simulink subsystem "PvtSubSys_LSM"  (R2020b)
settings: Solver=VariableStepAuto  StartTime=0.0  StopTime=10.0  RelTol=1e-3
values from neighbouring files (symbols this model uses):
  P_LSM_ALC_Enable = 0.0    [LSM_Parameter.sldd]
  P_LSM_DOP_C0_EN_Limit = 0.8    [LSM_Parameter.sldd]
  P_LSM_DOP_C0_out_Limit = 2.0    [LSM_Parameter.sldd]
  P_LSM_DOP_C1_EN_Limit : value not decoded    [LSM_Parameter.sldd]
  P_LSM_DOP_C1_out_Limit : value not decoded    [LSM_Parameter.sldd]
  P_LSM_DOP_C1AndC2_Lim_X : value not decoded    [LSM_Parameter.sldd]
  P_LSM_DOP_C2_EN_Limit : value not decoded    [LSM_Parameter.sldd]
  P_LSM_DOP_C2_out_Limit : value not decoded    [LSM_Parameter.sldd]
  P_LSM_DOP_In_Pre2Dop_Dis = 1.0    [LSM_Parameter.sldd]
  P_LSM_DOP_Out_Pre2Dop_Dis = 2.0    [LSM_Parameter.sldd]
  P_LSM_DOP_PreDis_X : value not decoded    [LSM_Parameter.sldd]
  P_LSM_DOP_PreDis_Y : value not decoded    [LSM_Parameter.sldd]
  P_LSM_DOPValid_CheckTime = 0.06    [LSM_Parameter.sldd]
  P_LSM_DoubleLine_Curr2Cent_Dislimit = 0.5    [LSM_Parameter.sldd]
  P_LSM_DoubleLine_Dop2Cent_Dislimit = 0.5    [LSM_Parameter.sldd]
  P_LSM_DoubleLine_DOPOut_C1 : value not decoded    [LSM_Parameter.sldd]
  P_LSM_DoubleLine_Pre2Cent_Dislimit = 1.0    [LSM_Parameter.sldd]
  P_LSM_IFV2CenterAxis = 0.0    [LSM_Parameter.sldd]
  P_LSM_IFV2RearAxis = 0.0    [LSM_Parameter.sldd]
  P_LSM_LineSTD_Limit = 0.15    [LSM_Parameter.sldd]
  P_LSM_NOH_Switch = 0.0    [LSM_Parameter.sldd]
  P_LSM_Pre_t = 0.0    [LSM_Parameter.sldd]
  P_LSM_SingleLine_Cent2Edge_Dislimit = 100.0    [LSM_Parameter.sldd]
  P_LSM_SingleLine_Curr2Cent_Dislimit = 0.2    [LSM_Parameter.sldd]
  P_LSM_SingleLine_Dop2Cent_Dislimit = 0.2    [LSM_Parameter.sldd]
  P_LSM_SingleLine_DOPOut_C1 : value not decoded    [LSM_Parameter.sldd]
  P_LSM_SingleLine_Pre2Cent_Dislimit = 0.5    [LSM_Parameter.sldd]
undefined symbols (not defined in the file or in its folder): P_LSM_LineWijCal_C12, P_LSM_LineWijCal_C13, P_LSM_PosLineLcFac
libraries: simulink x92, TrueDurationTime x2
(part 1 of 9)
settings Model: Creator=GW00232905  LastModifiedBy=GW00232905

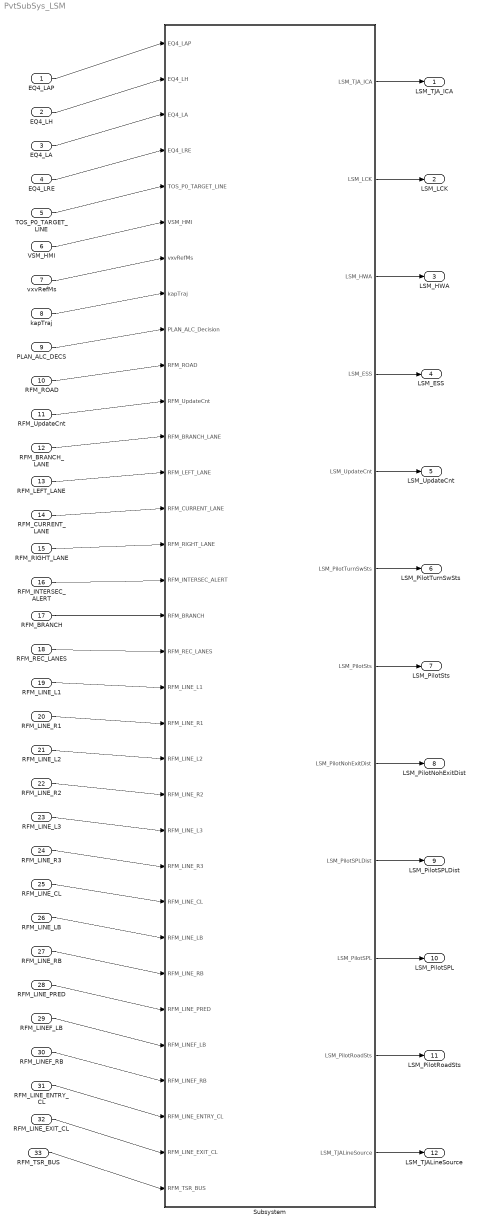
== system PvtSubSys_LSM ==
  EQ4_LAP : Inport  Description=预留  OutDataTypeStr=Bus: EQ4_LAP_BUS  PortDimensions=1  BusOutputAsStruct=on
  EQ4_LH : Inport  Description=|  Port=2  OutDataTypeStr=Bus: EQ4_LH_BUS  PortDimensions=1  BusOutputAsStruct=on
      | LH_Sync_ID	 	uint8		|		判断主车道线是否更新
      | LA_Lanes_Count		uint8		|		主车道线数量
      | LH_Availability_Stat  	uint8		|		主车道线是否可用
      | LH_Line_First_C0		single		m		主车道线第一段参数C0;曲线方程：y=c0+c1*x+c2*x^2+c3*x^3;
      | LH_Line_First_C1	         single		rad		主车道线第一段参数C1
      | LH_Line_First_C2	         single		1/m		主车道线第一段参数C2
      | LH_Line_First_C3	         single		1/m^2		主车道线第一段参数C3
      | LH_First_VR_Start	         single		m		主车道线第一段有效范围起点
      | LH_First_VR_End	         single		m		主车道线第一段有效范围终点
      | LH_lanemark_Type	         uint8		|		主车道线标记类型分类(实线，虚线等)
      | LH_DLM_Type	         uint8		|		主车道线双车道线标志
      | LH_Side	                   uint8		|		主车道线边界
      | LH_Marker_Width	         single		m		主车道线宽度
      | LH_Crossing	         uint8		|		判断是否跨越车道线
      | LH_Confidence	         uint8		|		主车道线置信度
      | LH_Color	                   uint8		|		主车道线颜色
      | LH_Line_Second_C0	          single		m		主车道线第二段参数C0;曲线方程：y=c0+c1*x+c2*x^2+c3*x^3
      | LH_Line_Second_C1	          single		rad		主车道线第二段参数C1
      | LH_Line_Second_C2	          single		1/m		主车道线第二段参数C2
      | LH_Line_Second_C3	          single		1/m^2		主车道线第二段参数C3
      | LH_Second_VR_Start	          single		m		主车道线第二段有效范围起点
      | LH_Second_VR_End	          single		m		主车道线第二段有效范围终点
  EQ4_LA : Inport  Description=|  Port=3  OutDataTypeStr=Bus: EQ4_LA_BUS  PortDimensions=1  BusOutputAsStruct=on
      | LA_Sync_ID		uint8		|		判断邻车道线是否更新
      | LA_Adjacent_Count		uint8		|		邻车道线数量		
      | LA_Availability_State	uint8		|		车道边界是否可用
      | LA_Line_C0		single		m		邻车道参数C0;曲线方程：y=c0+c1*x+c2*x^2+c3*x^3;
      | LA_Line_C1		single		rad		邻车道参数C1
      | LA_Line_C2		single		1/m		邻车道参数C2
      | LA_Line_C3		single		1/m^2		邻车道参数C3
      | LA_View_Range_Start	single		m		邻车道线有效范围起点
      | LA_View_Range_End	         single		m		邻车道线有效范围终点
      | LA_Lanemark_Type		uint8		|		邻车道线标记类型分类（实线，虚线等）
      | LA_DLM_Type		uint8		|		邻车道线双车道线标志
      | LA_Line_Side		uint8		|		车道标志相对于主车道的作用
      | LA_Marker_Width		single		m		车道线宽度
      | LA_Confidence		uint8		|		车道标志的置信度
  EQ4_LRE : Inport  Description=|  Port=4  OutDataTypeStr=Bus: EQ4_LRE_BUS  PortDimensions=1  BusOutputAsStruct=on
      | LRE_Sync_ID		uint8		|		判断边界车道线是否更新
      | LRE_Count		          uint8		|		边界车道线数量			
      | LRE_AvaiLREbility_State	uint8		|		边界车道线是否可用
      | LRE_Line_C0		single		m		边界车道线参数C0;曲线方程：y=c0+c1*x+c2*x^2+c3*x^3;
      | LRE_Line_C1		single		rad		边界车道线参数C1
      | LRE_Line_C2		single		1/m		边界车道线参数C2
      | LRE_Line_C3		single		1/m^2		边界车道线参数C3
      | LRE_View_Range_Start	single		m		边界车道线有效范围起点
      | LRE_View_Range_End	         single		m		边界车道线有效范围终点
      | LRE_Side			uint8		|		边界车道线标记
      | LRE_Confidence		uint8		|		边界车道线置信度
  TOS_P0_TARGET_LINE : Inport  Description=|  Port=5  OutDataTypeStr=Bus: TOS_P0_TARGET_LINE_BUS  PortDimensions=1  BusOutputAsStruct=on
      | OTL_Valid     uint8     |       OTL是否有效
      | OTL_C3        single    1/m^2   OTL参数C3;曲线方程：y=c0+c1*x+c2*x^2+c3*x^3
      | OTL_C2        single    1/m     OTL参数C2
      | OTL_C1        single    rad     OTL参数C1
      | OTL_C0        single    m       OTL参数C0
      | OTL_Range     single    m       OTL线有效范围
  VSM_HMI : Inport  Description=|  Port=6  OutDataTypeStr=Bus: VSM_HMI_BUS  PortDimensions=1  BusOutputAsStruct=on
      | ACC_ModeDisp    uint8    |   ACC仪表显示状态
      | HWASts          uint8    |   HWA功能状态
      | LCKSts          uint8    |   LCK功能状态
      | ESSSts          uint8    |   ESS功能状态
      | NOH_Sts         uint8    |   NOH功能状态
  vxvRefMs : Inport  Description=m/s|自车参考车速  Port=7  OutDataTypeStr=single  PortDimensions=1  BusOutputAsStruct=on
  kapTraj : Inport  Description=1/m|自车参考曲率  Port=8  OutDataTypeStr=single  PortDimensions=1  BusOutputAsStruct=on
  PLAN_ALC_DECS : Inport  Description=预留  Port=9  OutDataTypeStr=Bus: PLAN_ALC_DECS_BUS  PortDimensions=1  BusOutputAsStruct=on
  RFM_ROAD : Inport  Description=|  Port=10  OutDataTypeStr=Bus: RFM_ROAD_BUS  PortDimensions=1  BusOutputAsStruct=on
      | nLaneID                 uint8          |      自动驾驶车辆所在车道ID（从左往右）
      | nLaneNum                uint8          |      当前总车道数
      | dCurrentLaneWidth       single         m      本车道宽度
      | dLeftLaneWidth          single         m      左侧相邻，车道宽度
      | dRightLaneWidth         single         m      右侧相邻，车道宽度
      | bCurrentLaneFree        uint8          |      当前车道是否可行驶（freespace 可用）
      | fCurrentLaneFreeDis     single         m      当前可行驶距离
      | bLeftLaneFree           uint8          |      左侧车道是否可行驶（freespace 可用）
      | fLeftLaneFreeDis        single         m      左侧可行驶距离
      | bRightLaneFree          uint8          |      右侧车道是否可行驶（freespace 可用）
      | fRighLaneFreeDis        single         m      右侧可行驶距离
      | b_toll                  uint8          |      前方是否有收费站
      | f_toll_distance         single         m      到收费站距离
      | b_tunnel                uint8          |      车辆是否在隧道
      | f_tunnel_distance       single         m      到隧道的距离
      | b_bridge                uint8          |      车辆是否在桥梁上
      | f_bridge_distance       single         m      到桥梁的距离
      | b_traffic_jam           uint8          |      前方是否有交通拥堵
      | f_distance_to_jam       single         m      到交通拥堵点的距离
      | b_traffic_accident      uint8          |      前方是否发生交通事故
      | f_distance_to_accident  single         m      到交通事故发生点的距离
      | en_weather              uint8          |      天气情况
      | i_mapvalid              uint8          |      V2、V3有效性
      | i_on_nav_path           uint8          |      是否行驶在导航路径上
  RFM_UpdateCnt : Inport  Description=|模块更新计数器  Port=11  OutDataTypeStr=uint32  PortDimensions=1  BusOutputAsStruct=on
  RFM_BRANCH_LANE : Inport  Description=预留  Port=12  OutDataTypeStr=Bus: RFM_LANE_BUS  PortDimensions=1  BusOutputAsStruct=on
  RFM_LEFT_LANE : Inport  Description=预留  Port=13  OutDataTypeStr=Bus: RFM_LANE_BUS  PortDimensions=1  BusOutputAsStruct=on
  RFM_CURRENT_LANE : Inport  Description=|  Port=14  OutDataTypeStr=Bus: RFM_LANE_BUS  PortDimensions=1  BusOutputAsStruct=on
      | b_is_avalible         uint8         |          车道是否可用
      | en_lane_type          uint8         |          当前车道类型
      | i_speed_max           uint8         kmph       当前限速
      | f_spd_change_dis      single        m          前方限速变化距离
      | i_change_spd_max      uint8         kmph       限速变化后的值
      | f_width               single        m          车道宽度
      | b_vanish_valid        uint8         |          当前是否为消失车道
      | f_vanish_pt_dis       single        m          到消失点的距离
  RFM_RIGHT_LANE : Inport  Description=预留  Port=15  OutDataTypeStr=Bus: RFM_LANE_BUS  PortDimensions=1  BusOutputAsStruct=on
  RFM_INTERSEC_ALERT : Inport  Description=|  Port=16  OutDataTypeStr=Bus: RFM_INTERSEC_ALERT_BUS  PortDimensions=1  BusOutputAsStruct=on
      | b_is_available    uint8      |  是否可用:0：否 1：是前方1000m有路口时给出true
      | f_distance        single     m  到最近路口距离
      | en_direction      uint8      |    unknown：0X0,左驶出：0x1,右驶出：0x2,左直行：0x3,右直行：0x4,驶入：0x5"
      | en_type           uint8      |    unknown：0X0,高速到匝道（汇出）：0X1,高速到高速（汇出）：0X2,匝道到匝道（汇出）：0X3,匝道汇入高速（汇入）：0X4,前方有匝道汇入：0x5
  RFM_BRANCH : Inport  Description=预留  Port=17  OutDataTypeStr=Bus: RFM_BRANCH_BUS  PortDimensions=1  BusOutputAsStruct=on
  RFM_REC_LANES : Inport  Description=|  Port=18  OutDataTypeStr=Bus: RFM_REC_LANES_BUS  PortDimensions=1  BusOutputAsStruct=on
      | i_rec_lanes_num     uint8     |       推荐行驶车道处车道总数
      | i_rec_lanes         uint8     |       推荐行驶车道数组（最多8个元素）
  RFM_LINE_L1 : Inport  Description=|  Port=19  OutDataTypeStr=Bus: RFM_LINE_BUS  PortDimensions=1  BusOutputAsStruct=on
      | bIsLineExist      uint8          |    表示车道线有无，2为有，1为无
      | dC0V              single         m    车辆坐标系下，车道线参数C0
      | dC1V              single         |    车辆坐标系下，车道线参数C1
      | dC2V              single         |    车辆坐标系下，车道线参数C2
      | dC3V              single         |    车辆坐标系下，车道线参数C3
      | dLaneWidth        single         m    车道线宽度
      | eLineType         uint8          |    车道线线型（普通、实线、虚线、路牙...）"
      | dDisStart         single         m    车道线前方，起点长度
      | dDisFront         single         m    车道线前方，有效长度
      | dQuality          single         |    车道线质量信息
      | eColour           uint8          |    车道线颜色
      | eFuType           uint8          |    车道线融合状态（无、摄像头、地图、摄像头融合地图、预留）
      | nTrackAge         uint8          |    车道线预测周期数（未预测时为0）
  RFM_LINE_R1 : Inport  Description=|  Port=20  OutDataTypeStr=Bus: RFM_LINE_BUS  PortDimensions=1  BusOutputAsStruct=on
      | bIsLineExist      uint8          |    表示车道线有无，2为有，1为无
      | dC0V              single         m    车辆坐标系下，车道线参数C0
      | dC1V              single         |    车辆坐标系下，车道线参数C1
      | dC2V              single         |    车辆坐标系下，车道线参数C2
      | dC3V              single         |    车辆坐标系下，车道线参数C3
      | dLaneWidth        single         m    车道线宽度
      | eLineType         uint8          |    车道线线型（普通、实线、虚线、路牙...）"
      | dDisStart         single         m    车道线前方，起点长度
      | dDisFront         single         m    车道线前方，有效长度
      | dQuality          single         |    车道线质量信息
      | eColour           uint8          |    车道线颜色
      | eFuType           uint8          |    车道线融合状态（无、摄像头、地图、摄像头融合地图、预留）
      | nTrackAge         uint8          |    车道线预测周期数（未预测时为0）
  RFM_LINE_L2 : Inport  Description=|  Port=21  OutDataTypeStr=Bus: RFM_LINE_BUS  PortDimensions=1  BusOutputAsStruct=on
      | bIsLineExist      uint8          |    表示车道线有无，2为有，1为无
      | dC0V              single         m    车辆坐标系下，车道线参数C0
      | dC1V              single         |    车辆坐标系下，车道线参数C1
      | dC2V              single         |    车辆坐标系下，车道线参数C2
      | dC3V              single         |    车辆坐标系下，车道线参数C3
      | dLaneWidth        single         m    车道线宽度
      | eLineType         uint8          |    车道线线型（普通、实线、虚线、路牙...）"
      | dDisStart         single         m    车道线前方，起点长度
      | dDisFront         single         m    车道线前方，有效长度
      | dQuality          single         |    车道线质量信息
      | eColour           uint8          |    车道线颜色
      | eFuType           uint8          |    车道线融合状态（无、摄像头、地图、摄像头融合地图、预留）
      | nTrackAge         uint8          |    车道线预测周期数（未预测时为0）
  RFM_LINE_R2 : Inport  Description=|  Port=22  OutDataTypeStr=Bus: RFM_LINE_BUS  PortDimensions=1  BusOutputAsStruct=on
      | bIsLineExist      uint8          |    表示车道线有无，2为有，1为无
      | dC0V              single         m    车辆坐标系下，车道线参数C0
      | dC1V              single         |    车辆坐标系下，车道线参数C1
      | dC2V              single         |    车辆坐标系下，车道线参数C2
      | dC3V              single         |    车辆坐标系下，车道线参数C3
      | dLaneWidth        single         m    车道线宽度
      | eLineType         uint8          |    车道线线型（普通、实线、虚线、路牙...）"
      | dDisStart         single         m    车道线前方，起点长度
      | dDisFront         single         m    车道线前方，有效长度
      | dQuality          single         |    车道线质量信息
      | eColour           uint8          |    车道线颜色
      | eFuType           uint8          |    车道线融合状态（无、摄像头、地图、摄像头融合地图、预留）
      | nTrackAge         uint8          |    车道线预测周期数（未预测时为0）
  RFM_LINE_L3 : Inport  Description=预留  Port=23  OutDataTypeStr=Bus: RFM_LINE_BUS  PortDimensions=1  BusOutputAsStruct=on
  RFM_LINE_R3 : Inport  Description=预留  Port=24  OutDataTypeStr=Bus: RFM_LINE_BUS  PortDimensions=1  BusOutputAsStruct=on
  RFM_LINE_CL : Inport  Description=预留  Port=25  OutDataTypeStr=Bus: RFM_LINE_BUS  PortDimensions=1  BusOutputAsStruct=on
  RFM_LINE_LB : Inport  Description=预留  Port=26  OutDataTypeStr=Bus: RFM_LINE_BUS  PortDimensions=1  BusOutputAsStruct=on
  RFM_LINE_RB : Inport  Description=预留  Port=27  OutDataTypeStr=Bus: RFM_LINE_BUS  PortDimensions=1  BusOutputAsStruct=on
  RFM_LINE_PRED : Inport  Description=|  Port=28  OutDataTypeStr=Bus: RFM_LINE_BUS  PortDimensions=1  BusOutputAsStruct=on
      | bIsLineExist      uint8          |    表示车道线有无，2为有，1为无
      | dC0V              single         m    车辆坐标系下，车道线参数C0
      | dC1V              single         |    车辆坐标系下，车道线参数C1
      | dC2V              single         |    车辆坐标系下，车道线参数C2
      | dC3V              single         |    车辆坐标系下，车道线参数C3
      | dLaneWidth        single         m    车道线宽度
      | eLineType         uint8          |    车道线线型（普通、实线、虚线、路牙...）"
      | dDisStart         single         m    车道线前方，起点长度
      | dDisFront         single         m    车道线前方，有效长度
      | dQuality          single         |    车道线质量信息
      | eColour           uint8          |    车道线颜色
      | eFuType           uint8          |    车道线融合状态（无、摄像头、地图、摄像头融合地图、预留）
      | nTrackAge         uint8          |    车道线预测周期数（未预测时为0）
  RFM_LINEF_LB : Inport  Description=预留  Port=29  OutDataTypeStr=Bus: RFM_LINE_BUS  PortDimensions=1  BusOutputAsStruct=on
  RFM_LINEF_RB : Inport  Description=预留  Port=30  OutDataTypeStr=Bus: RFM_LINE_BUS  PortDimensions=1  BusOutputAsStruct=on
  RFM_LINE_ENTRY_CL : Inport  Description=|  Port=31  OutDataTypeStr=Bus: RFM_LINE_BUS  PortDimensions=1  BusOutputAsStruct=on
      | bIsLineExist      uint8          |    表示车道线有无，2为有，1为无
      | dC0V              single         m    车辆坐标系下，车道线参数C0
      | dC1V              single         |    车辆坐标系下，车道线参数C1
      | dC2V              single         |    车辆坐标系下，车道线参数C2
      | dC3V              single         |    车辆坐标系下，车道线参数C3
      | dLaneWidth        single         m    车道线宽度
      | eLineType         uint8          |    车道线线型（普通、实线、虚线、路牙...）"
      | dDisStart         single         m    车道线前方，起点长度
      | dDisFront         single         m    车道线前方，有效长度
      | dQuality          single         |    车道线质量信息
      | eColour           uint8          |    车道线颜色
      | eFuType           uint8          |    车道线融合状态（无、摄像头、地图、摄像头融合地图、预留）
      | nTrackAge         uint8          |    车道线预测周期数（未预测时为0）
  RFM_LINE_EXIT_CL : Inport  Description=|  Port=32  OutDataTypeStr=Bus: RFM_LINE_BUS  PortDimensions=1  BusOutputAsStruct=on
      | bIsLineExist      uint8          |    表示车道线有无，2为有，1为无
      | dC0V              single         m    车辆坐标系下，车道线参数C0
      | dC1V              single         |    车辆坐标系下，车道线参数C1
      | dC2V              single         |    车辆坐标系下，车道线参数C2
      | dC3V              single         |    车辆坐标系下，车道线参数C3
      | dLaneWidth        single         m    车道线宽度
      | eLineType         uint8          |    车道线线型（普通、实线、虚线、路牙...）"
      | dDisStart         single         m    车道线前方，起点长度
      | dDisFront         single         m    车道线前方，有效长度
      | dQuality          single         |    车道线质量信息
      | eColour           uint8          |    车道线颜色
      | eFuType           uint8          |    车道线融合状态（无、摄像头、地图、摄像头融合地图、预留）
      | nTrackAge         uint8          |    车道线预测周期数（未预测时为0）
  RFM_TSR_BUS : Inport  Description=|  Port=33  OutDataTypeStr=Bus: RFM_TSR_BUS
      | RoadType              uint8     |     指示导航检测到的车辆当前行驶位置的行驶类型(HUT)
      | VehInLeftmostLane     uint8     |     指示是否在最左侧车道
      | VehInRightmostLane    uint8     |     指示是否在最右侧车道
      | SPL_LaneChanged       uint8     |     指示是否发生变道以及变道向哪个方向
  Subsystem : Subsystem
  LSM_TJA_ICA : Outport  Description=|  OutDataTypeStr=Bus: LSM_TJA_ICA_BUS  PortDimensions=1  BusOutputAsStruct=on
      | TJALineValid	boolean		|		目标线有效性
      | TJALineC3	          single		1/m^2		TJA_ICA目标线参数C3;曲线方程：y=c0+c1*x+c2*x^2+c3*x^3;
      | TJALineC2	          single		1/m		TJA_ICA目标线参数C2
      | TJALineC1	          single		rad		TJA_ICA目标线参数C1
      | TJALineC0	          single		m		TJA_ICA目标线参数C0
      | TJARange		 single		m		目标线有效长度，基于车辆坐标系x轴正方向长度（>=0）
  LSM_LCK : Outport  Description=|  Port=2  OutDataTypeStr=Bus: LSM_LCK_BUS  PortDimensions=1  BusOutputAsStruct=on
      | LCKLineValid	  boolean		|		目标线有效性
      | LCKLineC3	           single		1/m^2		目标线参数C3;曲线方程：y=c0+c1*x+c2*x^2+c3*x^3;
      | LCKLineC2	           single		1/m		目标线参数C2
      | LCKLineC1        	  single		rad		目标线参数C1
      | LCKLineC0	           single		m		目标线参数C0
      | LCKRange	           single		m		目标线有效长度，基于车辆坐标系x轴正方向长度（>=0）
  LSM_HWA : Outport  Description=|  Port=3  OutDataTypeStr=Bus: LSM_HWA_BUS  PortDimensions=1  BusOutputAsStruct=on
      | HWALineValid	boolean		|		HWA本车道目标线是否有效
      | HWALineC3	         single		1/m^2		"y = C3*x^3 + C2*x^2 +C1*x + C0"
      | HWALineC2	         single		1/m		"y = C3*x^3 + C2*x^2 +C1*x + C0"
      | HWALineC1	         single		rad		"y = C3*x^3 + C2*x^2 +C1*x + C0"
      | HWALineC0	         single		m		"y = C3*x^3 + C2*x^2 +C1*x + C0"
      | HWARange	         single		m		目标线有效距离
      | HWALeLineValid	boolean		|		HWA左车道目标线是否有效
      | HWALeLineC3	single		1/m^2		"y = C3*x^3 + C2*x^2 +C1*x + C0"
      | HWALeLineC2	single		1/m		"y = C3*x^3 + C2*x^2 + C1*x + C0"
      | HWALeLineC1	single		rad		"y = C3*x^3 + C2*x^2 +C1*x + C0"
      | HWALeLineC0	single		m		"y = C3*x^3 + C2*x^2 +C1*x + C0"
      | HWALeRange	single		m		目标线有效距离
      | HWARiLineValid	boolean		|		HWA右车道目标线是否有效
      | HWARiLineC3	single		1/m^2		"y = C3*x^3 + C2*x^2 +C1*x + C0"
      | HWARiLineC2	single		1/m		"y = C3*x^3 + C2*x^2 +C1*x + C0"
      | HWARiLineC1	single		rad		"y = C3*x^3 + C2*x^2 +C1*x + C0"
      | HWARiLineC0	single		m		"y = C3*x^3 + C2*x^2 +C1*x + C0"
      | HWARiRange	single		m		目标线有效距离
      | dyDiff		uint8		|		横向距离与目标车道中心线横向偏差
      | HeadAngDiff	uint8		|		航向角与目标车道中心线偏差
      | MLeLane		uint8		|		是否在最左侧车道
      | RoadWidth	         uint8		|		道路宽度
      | LeftLaneChange	uint8		|		是否自车左换道
      | RightLaneChange	uint8		|		是否自车右换道
      | SingleLineLost_b	boolean		|		本车道单侧车道线丢失
      | DoubleLineLost_b	boolean		|		本车道双侧车道线丢失
      | MRiLane		boolean		|		是否在最右侧车道
      | MrcStopLane	uint8		|		紧急停车道使能条件
      | HWALeLineVirtual	boolean		|		左车道中心线是否是虚拟中心线
      | HWARiLineVirtual	boolean		|		右车道中心线是否是虚拟中心线
      | LeLineLcAvailable	boolean		|		本车道左线是否可用（即为虚线或实线）
      | RiLineLcAvailable	boolean		|		本车道右线是否可用（即为虚线或实线）
  LSM_ESS : Outport  Description=|  Port=4  OutDataTypeStr=Bus: LSM_ESS_BUS  PortDimensions=1  BusOutputAsStruct=on
      | ESSLineValid	boolean		|		目标线是否有效
      | ESSLineC3	         single		1/m^2		"y = C3*x^3 + C2*x^2 +C1*x + C0"
      | ESSLineC2	         single		1/m		"y = C3*x^3 + C2*x^2 +C1*x + C0"
      | ESSLineC1	         single		rad		"y = C3*x^3 + C2*x^2 +C1*x + C0"
      | ESSLineC0	         single		m		"y = C3*x^3 + C2*x^2 +C1*x + C0"
      | ESSRange		single		m		目标线有效距离
      | ESSLeLineValid	boolean		|		目标线是否有效
      | ESSLeLineC3	single		1/m^2		"y = C3*x^3 + C2*x^2 +C1*x + C0"
      | ESSLeLineC2	single		1/m		"y = C3*x^3 + C2*x^2 +C1*x + C0"
      | ESSLeLineC1	single		rad		"y = C3*x^3 + C2*x^2 +C1*x + C0"
      | ESSLeLineC0	single		m		"y = C3*x^3 + C2*x^2 +C1*x + C0"
      | ESSLeRange	single		m		目标线有效距离
      | ESSRiLineValid	boolean		|		目标线是否有效
      | ESSRiLineC3	single		1/m^2		"y = C3*x^3 + C2*x^2 +C1*x + C0"
      | ESSRiLineC2	single		1/m		"y = C3*x^3 + C2*x^2 +C1*x + C0"
      | ESSRiLineC1	single		rad		"y = C3*x^3 + C2*x^2 +C1*x + C0"
      | ESSRiLineC0	single		m		"y = C3*x^3 + C2*x^2 +C1*x + C0"
      | ESSRiRange	single		m		目标线有效距离
  LSM_UpdateCnt : Outport  Description=|LSM模块计数器  Port=5  OutDataTypeStr=uint32  PortDimensions=1  BusOutputAsStruct=on
  LSM_PilotTurnSwSts : Outport  Description=|给Plan模块的换道请求  Port=6  OutDataTypeStr=uint8  PortDimensions=1  BusOutputAsStruct=on
  LSM_PilotSts : Outport  Description=|Pilot HWA使能条件  Port=7  OutDataTypeStr=uint8  PortDimensions=1  BusOutputAsStruct=on
  LSM_PilotNohExitDist : Outport  Description=m|距离高速公路出口的距离  Port=8  OutDataTypeStr=uint16  PortDimensions=1  BusOutputAsStruct=on
  LSM_PilotSPLDist : Outport  Description=m|HMI接收（预留）  Port=9  OutDataTypeStr=uint16  PortDimensions=1  BusOutputAsStruct=on
  LSM_PilotSPL : Outport  Description=km/h|汇出时的速度限制  Port=10  OutDataTypeStr=uint8  PortDimensions=1  BusOutputAsStruct=on
  LSM_PilotRoadSts : Outport  Description=|NOA道路区域类型  Port=11  OutDataTypeStr=uint8  PortDimensions=1  BusOutputAsStruct=on
  LSM_TJALineSource : Outport  Description=|DOP到车道线切换  Port=12  OutDataTypeStr=uint8  PortDimensions=1  BusOutputAsStruct=on
  wires:
  RFM_LINE_L3/1 -> Subsystem/23(RFM_LINE_L3)
  RFM_RIGHT_LANE/1 -> Subsystem/15(RFM_RIGHT_LANE)
  EQ4_LA/1 -> Subsystem/3(EQ4_LA)
  Subsystem/7(LSM_PilotSts) -> LSM_PilotSts/1
  EQ4_LRE/1 -> Subsystem/4(EQ4_LRE)
  EQ4_LH/1 -> Subsystem/2(EQ4_LH)
  RFM_TSR_BUS/1 -> Subsystem/33(RFM_TSR_BUS)
  Subsystem/12(LSM_TJALineSource) -> LSM_TJALineSource/1
  Subsystem/1(LSM_TJA_ICA) -> LSM_TJA_ICA/1
  RFM_LINEF_RB/1 -> Subsystem/30(RFM_LINEF_RB)
  Subsystem/2(LSM_LCK) -> LSM_LCK/1
  RFM_LINE_CL/1 -> Subsystem/25(RFM_LINE_CL)
  RFM_LINE_RB/1 -> Subsystem/27(RFM_LINE_RB)
  RFM_LINE_R3/1 -> Subsystem/24(RFM_LINE_R3)
  PLAN_ALC_DECS/1 -> Subsystem/9(PLAN_ALC_Decision)
  RFM_ROAD/1 -> Subsystem/10(RFM_ROAD)
  Subsystem/10(LSM_PilotSPL) -> LSM_PilotSPL/1
  RFM_UpdateCnt/1 -> Subsystem/11(RFM_UpdateCnt)
  RFM_LINE_L1/1 -> Subsystem/19(RFM_LINE_L1)
  Subsystem/6(LSM_PilotTurnSwSts) -> LSM_PilotTurnSwSts/1
  Subsystem/8(LSM_PilotNohExitDist) -> LSM_PilotNohExitDist/1
  RFM_LINEF_LB/1 -> Subsystem/29(RFM_LINEF_LB)
  RFM_INTERSEC_ALERT/1 -> Subsystem/16(RFM_INTERSEC_ALERT)
  RFM_CURRENT_LANE/1 -> Subsystem/14(RFM_CURRENT_LANE)
  kapTraj/1 -> Subsystem/8(kapTraj)
  VSM_HMI/1 -> Subsystem/6(VSM_HMI)
  TOS_P0_TARGET_LINE/1 -> Subsystem/5(TOS_P0_TARGET_LINE)
  Subsystem/9(LSM_PilotSPLDist) -> LSM_PilotSPLDist/1
  EQ4_LAP/1 -> Subsystem/1(EQ4_LAP)
  RFM_LINE_LB/1 -> Subsystem/26(RFM_LINE_LB)
  RFM_LINE_ENTRY_CL/1 -> Subsystem/31(RFM_LINE_ENTRY_CL)
  Subsystem/4(LSM_ESS) -> LSM_ESS/1
  vxvRefMs/1 -> Subsystem/7(vxvRefMs)
  RFM_LINE_L2/1 -> Subsystem/21(RFM_LINE_L2)
  RFM_LINE_R2/1 -> Subsystem/22(RFM_LINE_R2)
  RFM_LINE_PRED/1 -> Subsystem/28(RFM_LINE_PRED)
  Subsystem/5(LSM_UpdateCnt) -> LSM_UpdateCnt/1
  Subsystem/11(LSM_PilotRoadSts) -> LSM_PilotRoadSts/1
  RFM_BRANCH_LANE/1 -> Subsystem/12(RFM_BRANCH_LANE)
  Subsystem/3(LSM_HWA) -> LSM_HWA/1
  RFM_LINE_EXIT_CL/1 -> Subsystem/32(RFM_LINE_EXIT_CL)
  RFM_BRANCH/1 -> Subsystem/17(RFM_BRANCH)
  RFM_REC_LANES/1 -> Subsystem/18(RFM_REC_LANES)
  RFM_LINE_R1/1 -> Subsystem/20(RFM_LINE_R1)
  RFM_LEFT_LANE/1 -> Subsystem/13(RFM_LEFT_LANE)

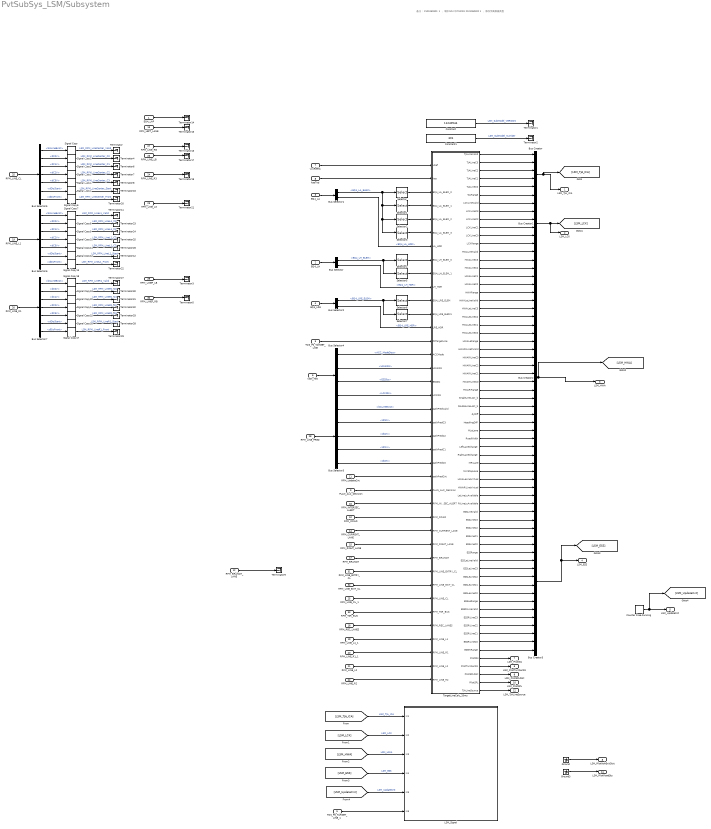
== system PvtSubSys_LSM/Subsystem ==
  note: 备注：
      | 2101060301:
      | 1、增加NOA中PilotSts
      | 2101060302
      | 1、修改字典数据类型
  EQ4_LAP : Inport
  EQ4_LH : Inport  Port=2  OutDataTypeStr=Bus: EQ4_LH_BUS  PortDimensions=1  BusOutputAsStruct=on
  EQ4_LA : Inport  Port=3  OutDataTypeStr=Bus: EQ4_LA_BUS  PortDimensions=1  BusOutputAsStruct=on
  EQ4_LRE : Inport  Port=4  OutDataTypeStr=Bus: EQ4_LRE_BUS  PortDimensions=1  BusOutputAsStruct=on
  TOS_P0_TARGET_LINE : Inport  Port=5  OutDataTypeStr=Bus: TOS_P0_TARGET_LINE_BUS  PortDimensions=1  BusOutputAsStruct=on
  VSM_HMI : Inport  Port=6  OutDataTypeStr=Bus: VSM_HMI_BUS  PortDimensions=1  BusOutputAsStruct=on
  vxvRefMs : Inport  Port=7  OutDataTypeStr=single  PortDimensions=1
  kapTraj : Inport  Port=8  OutDataTypeStr=single  PortDimensions=1
  PLAN_ALC_Decision : Inport  Port=9
  RFM_ROAD : Inport  Port=10  OutDataTypeStr=Bus: RFM_ROAD_BUS  PortDimensions=1  BusOutputAsStruct=on
  RFM_UpdateCnt : Inport  Port=11  OutDataTypeStr=uint32  PortDimensions=1  BusOutputAsStruct=on
  RFM_BRANCH_LANE : Inport  Port=12
  RFM_LEFT_LANE : Inport  Port=13
  RFM_CURRENT_LANE : Inport  Port=14
  RFM_RIGHT_LANE : Inport  Port=15
  RFM_INTERSEC_ALERT : Inport  Port=16
  RFM_BRANCH : Inport  Port=17
  RFM_REC_LANES : Inport  Port=18
  RFM_LINE_L1 : Inport  Port=19
  RFM_LINE_R1 : Inport  Port=20
  RFM_LINE_L2 : Inport  Port=21
  RFM_LINE_R2 : Inport  Port=22
  RFM_LINE_L3 : Inport  Port=23
  RFM_LINE_R3 : Inport  Port=24
  RFM_LINE_CL : Inport  Port=25
  RFM_LINE_LB : Inport  Port=26
  RFM_LINE_RB : Inport  Port=27
  RFM_LINE_PRED : Inport  Port=28  OutDataTypeStr=Bus: RFM_LINE_BUS  PortDimensions=1  BusOutputAsStruct=on
  RFM_LINEF_LB : Inport  Port=29
  RFM_LINEF_RB : Inport  Port=30
  RFM_LINE_ENTRY_CL : Inport  Port=31
  RFM_LINE_EXIT_CL : Inport  Port=32
  RFM_TSR_BUS : Inport  Port=33
  Bus Creator : BusCreator  Inputs=6
  Bus Creator1 : BusCreator  Inputs=6
  Bus Creator2 : BusCreator  Inputs=32
  Bus Creator3 : BusCreator  Inputs=18
  Bus Selector : BusSelector  OutputSignals=EQ4_LH_ELEM,EQ4_LH_HDR
  Bus Selector1 : BusSelector  OutputSignals=EQ4_LA_ELEM,EQ4_LA_HDR
  Bus Selector2 : BusSelector  OutputSignals=EQ4_LRE_ELEM,EQ4_LRE_HDR
  Bus Selector3 : BusSelector  OutputSignals=bIsLineExist,dC3V,dC2V,dC1V,dC0V
  Bus Selector4 : BusSelector  OutputSignals=ACC_ModeDisp,HWASts,ESSSts,LCKSts
  Bus Selector5 : BusSelector  OutputSignals=bIsLineExist,dC0V,dC1V,dC2V,dC3V,dDisStart,dDisFront
  Bus Selector6 : BusSelector  OutputSignals=bIsLineExist,dC0V,dC1V,dC2V,dC3V,dDisStart,dDisFront
  Bus Selector7 : BusSelector  OutputSignals=bIsLineExist,dC0V,dC1V,dC2V,dC3V,dDisStart,dDisFront
  Constant : Constant  Value=11240544  OutDataTypeStr=uint32
  Constant1 : Constant  Value=301  OutDataTypeStr=uint32
  Counter Free-Running : simulink/Sources/Counter Free-Running  NumBits=32  tsamp=-1
  Ground : Ground
  Ground3 : Ground
  LSM_Signal : Subsystem
  RFM_LINE_CL_1 : InportShadow  Port=25
  RFM_LINE_L1_1 : InportShadow  Port=19
  RFM_LINE_R1_1 : InportShadow  Port=20
  Selector : Selector  InputPortWidth=4  IndexOptions=Index vector (dialog)  Indices=1  OutputSizes=1
  Selector1 : Selector  InputPortWidth=4  IndexOptions=Index vector (dialog)  Indices=2  OutputSizes=1
  Selector2 : Selector  InputPortWidth=4  IndexOptions=Index vector (dialog)  Indices=3  OutputSizes=1
  Selector3 : Selector  InputPortWidth=4  IndexOptions=Index vector (dialog)  Indices=4  OutputSizes=1
  Selector4 : Selector  InputPortWidth=2  IndexOptions=Index vector (dialog)  Indices=1  OutputSizes=1
  Selector5 : Selector  InputPortWidth=2  IndexOptions=Index vector (dialog)  Indices=2  OutputSizes=1
  Selector6 : Selector  InputPortWidth=2  IndexOptions=Index vector (dialog)  Indices=1  OutputSizes=1
  Selector7 : Selector  InputPortWidth=2  IndexOptions=Index vector (dialog)  Indices=2  OutputSizes=1
  Signal Copy{,1..20} (21 alike) : SignalConversion  OverrideOpt=off
  TOS_P0_TARGET_LINE_1 : InportShadow  Port=5  OutDataTypeStr=Bus: TOS_P0_TARGET_LINE_BUS  PortDimensions=1  BusOutputAsStruct=on
  TargetLineCalc_20ms : Subsystem
  Terminator{,1..9,11..17,19..33} (32 alike) : Terminator
  LSM_TJA_ICA : Outport  OutDataTypeStr=Bus: LSM_TJA_ICA_BUS  PortDimensions=1  BusOutputAsStruct=on
  LSM_LCK : Outport  Port=2  OutDataTypeStr=Bus: LSM_LCK_BUS  PortDimensions=1  BusOutputAsStruct=on
  LSM_HWA : Outport  Port=3  OutDataTypeStr=Bus: LSM_HWA_BUS  PortDimensions=1  BusOutputAsStruct=on
  LSM_ESS : Outport  Port=4  OutDataTypeStr=Bus: LSM_ESS_BUS  PortDimensions=1  BusOutputAsStruct=on
  LSM_UpdateCnt : Outport  Port=5  OutDataTypeStr=uint32  PortDimensions=1  BusOutputAsStruct=on
  LSM_PilotTurnSwSts : Outport  Port=6
  LSM_PilotSts : Outport  Port=7
  LSM_PilotNohExitDist : Outport  Port=8
  LSM_PilotSPLDist : Outport  Port=9
  LSM_PilotSPL : Outport  Port=10
  LSM_PilotRoadSts : Outport  Port=11
  LSM_TJALineSource : Outport  Port=12
  wires:
  [LSM_HWA] -> LSM_Signal/3(In3)  "LSM_HWA"
  Signal Copy12/1 -> Terminator12/1  "LSM_RFM_LineL1_Start"
  Bus Creator/1 -> LSM_TJA_ICA/1, [LSM_TJA_ICA]
  Bus Selector5/4 -> Signal Copy3/1  "<dC2V>"
  Counter Free-Running/1 -> LSM_UpdateCnt/1, [LSM_UpdateCnt]
  TargetLineCalc_20ms/54(ESSLeLineC1) -> Bus Creator3/10
  RFM_RIGHT_LANE/1 -> TargetLineCalc_20ms/29(RFM_RIGHT_LANE)
  TargetLineCalc_20ms/12(LCKRange) -> Bus Creator1/6
  TargetLineCalc_20ms/66(PilotSPL) -> LSM_PilotSPL/1
  Bus Selector5/2 -> Signal Copy1/1  "<dC0V>"
  Bus Selector3/4 -> TargetLineCalc_20ms/22(pathPredC1)  "<dC1V>"
  TargetLineCalc_20ms/25(HWARiLineRValid) -> Bus Creator2/13
  Bus Selector3/2 -> TargetLineCalc_20ms/20(pathPredC3)  "<dC3V>"
  TOS_P0_TARGET_LINE_1/1 -> LSM_Signal/6(In6)
  Selector2/1 -> TargetLineCalc_20ms/5(EQ4_LA_ELEM_2)
  Bus Selector1/1 -> Selector3/1, Selector2/1, Selector1/1, Selector/1  "<EQ4_LA_ELEM>"
  Signal Copy1/1 -> Terminator4/1  "LSM_RFM_LineCenter_C0"
  Signal Copy8/1 -> Terminator23/1  "LSM_RFM_LineL1_C0"
  RFM_INTERSEC_ALERT/1 -> TargetLineCalc_20ms/26(RFM_INTERSEC_ALERT)
  TargetLineCalc_20ms/55(ESSLeLineC0) -> Bus Creator3/11
  RFM_LINE_LB/1 -> Terminator17/1
  TargetLineCalc_20ms/35(MLeLane) -> Bus Creator2/23
  Selector5/1 -> TargetLineCalc_20ms/9(EQ4_LH_ELEM_1)
  Bus Selector7/1 -> Signal Copy18/1  "<bIsLineExist>"
  RFM_LINE_CL/1 -> Bus Selector5/1
  Signal Copy18/1 -> Terminator27/1  "LSM_RFM_LineR1_Valid"
  Ground3/1 -> LSM_PilotRoadSts/1
  Selector4/1 -> TargetLineCalc_20ms/8(EQ4_LH_ELEM_0)
  Bus Selector7/4 -> Signal Copy14/1  "<dC2V>"
  Bus Selector3/3 -> TargetLineCalc_20ms/21(pathPredC2)  "<dC2V>"
  TargetLineCalc_20ms/21(HWALeLineC2) -> Bus Creator2/9
  Bus Selector7/2 -> Signal Copy19/1  "<dC0V>"
  EQ4_LAP/1 -> Terminator14/1
  Bus Selector2/1 -> Selector7/1, Selector6/1  "<EQ4_LRE_ELEM>"
  TargetLineCalc_20ms/13(HWALineValid) -> Bus Creator2/1
  kapTraj/1 -> TargetLineCalc_20ms/2(kap)
  Constant/1 -> Terminator1/1  "LSM_SubModel_VERSION"
  TargetLineCalc_20ms/58(ESSRiLineC3) -> Bus Creator3/14
  RFM_TSR_BUS/1 -> TargetLineCalc_20ms/34(RFM_TSR_BUS)
  RFM_LINE_ENTRY_CL/1 -> TargetLineCalc_20ms/31(RFM_LINE_ENTRY_CL)
  TargetLineCalc_20ms/17(HWALineC0) -> Bus Creator2/5
  Bus Selector7/3 -> Signal Copy20/1  "<dC1V>"
  RFM_CURRENT_LANE/1 -> TargetLineCalc_20ms/28(RFM_CURRENT_LANE)
  TargetLineCalc_20ms/24(HWALeRange) -> Bus Creator2/12
  TargetLineCalc_20ms/42(HWARiLineVirtual) -> Bus Creator2/30
  RFM_LINE_R1/1 -> Bus Selector7/1
  Signal Copy4/1 -> Terminator8/1  "LSM_RFM_LineCenter_C3"
  Signal Copy11/1 -> Terminator26/1  "LSM_RFM_LineL1_C3"
  TargetLineCalc_20ms/36(RoadWidth) -> Bus Creator2/24
  TargetLineCalc_20ms/60(ESSRiLineC1) -> Bus Creator3/16
  TargetLineCalc_20ms/27(HWARiLineC2) -> Bus Creator2/15
  Bus Selector4/4 -> TargetLineCalc_20ms/18(LCKSts)  "<LCKSts>"
  RFM_LINE_R1_1/1 -> TargetLineCalc_20ms/37(RFM_LINE_R1)
  Signal Copy6/1 -> Terminator20/1  "LSM_RFM_LineCenter_Front"
  Selector6/1 -> TargetLineCalc_20ms/11(EQ4_LRE_ELEM)
  RFM_LINEF_LB/1 -> Terminator3/1
  RFM_BRANCH_LANE/1 -> Terminator9/1
  Signal Copy/1 -> Terminator/1  "LSM_RFM_LineCenter_Valid"
  TargetLineCalc_20ms/63(PilotSts) -> LSM_PilotSts/1
  RFM_LINE_CL_1/1 -> TargetLineCalc_20ms/33(RFM_LINE_CL)
  VSM_HMI/1 -> Bus Selector4/1
  Bus Selector/2 -> TargetLineCalc_20ms/10(LH_HDR)  "<EQ4_LH_HDR>"
  Bus Selector/1 -> Selector5/1, Selector4/1  "<EQ4_LH_ELEM>"
  TargetLineCalc_20ms/43(LeLineLcAvailable) -> Bus Creator2/31
  TargetLineCalc_20ms/30(HWARiRange) -> Bus Creator2/18
  RFM_LINE_R3/1 -> Terminator19/1
  RFM_LINE_RB/1 -> Terminator13/1
  TargetLineCalc_20ms/65(PilotSPLDist) -> LSM_PilotSPLDist/1
  TargetLineCalc_20ms/49(ESSLineC0) -> Bus Creator3/5
  Bus Selector7/6 -> Signal Copy16/1  "<dDisStart>"
  TargetLineCalc_20ms/61(ESSRiLineC0) -> Bus Creator3/17
  RFM_LINE_PRED/1 -> Bus Selector3/1
  Bus Selector6/4 -> Signal Copy10/1  "<dC2V>"
  RFM_LINE_L1/1 -> Bus Selector6/1
  TargetLineCalc_20ms/52(ESSLeLineC3) -> Bus Creator3/8
  Signal Copy10/1 -> Terminator25/1  "LSM_RFM_LineL1_C2"
  TargetLineCalc_20ms/2(TJALineC3) -> Bus Creator/2
  Bus Selector6/3 -> Signal Copy9/1  "<dC1V>"
  TargetLineCalc_20ms/47(ESSLineC2) -> Bus Creator3/3
  Signal Copy7/1 -> Terminator11/1  "LSM_RFM_LineL1_Valid"
  [LSM_ESS] -> LSM_Signal/4(In4)  "LSM_ESS"
  TargetLineCalc_20ms/46(ESSLineC3) -> Bus Creator3/2
  Bus Selector1/2 -> TargetLineCalc_20ms/7(LA_HDR)  "<EQ4_LA_HDR>"
  TargetLineCalc_20ms/34(HeadAngDiff) -> Bus Creator2/22
  Signal Copy20/1 -> Terminator31/1  "LSM_RFM_LineR1_C1"
  Signal Copy5/1 -> Terminator16/1  "LSM_RFM_LineCenter_Start"
  Signal Copy9/1 -> Terminator24/1  "LSM_RFM_LineL1_C1"
  Signal Copy16/1 -> Terminator28/1  "LSM_RFM_LineR1_Start"
  Bus Selector3/1 -> TargetLineCalc_20ms/19(pathPredValid)  "<bIsLineExist>"
  Bus Selector4/3 -> TargetLineCalc_20ms/17(ESSSts)  "<ESSSts>"
  TargetLineCalc_20ms/15(HWALineC2) -> Bus Creator2/3
  EQ4_LH/1 -> Bus Selector/1
  RFM_BRANCH/1 -> TargetLineCalc_20ms/30(RFM_BRANCH)
  Bus Selector7/7 -> Signal Copy17/1  "<dDisFront>"
  TargetLineCalc_20ms/19(HWALeLineValid) -> Bus Creator2/7
  Signal Copy3/1 -> Terminator7/1  "LSM_RFM_LineCenter_C2"
  TargetLineCalc_20ms/50(ESSRange) -> Bus Creator3/6
  TargetLineCalc_20ms/10(LCKLineC1) -> Bus Creator1/4
  Selector3/1 -> TargetLineCalc_20ms/6(EQ4_LA_ELEM_3)
  TargetLineCalc_20ms/28(HWARiLineC1) -> Bus Creator2/16
  RFM_LINEF_RB/1 -> Terminator5/1
  Selector1/1 -> TargetLineCalc_20ms/4(EQ4_LA_ELEM_1)
  Bus Selector5/5 -> Signal Copy4/1  "<dC3V>"
  TargetLineCalc_20ms/31(SingleLineLost_b) -> Bus Creator2/19
  TargetLineCalc_20ms/37(LeftLaneChange) -> Bus Creator2/25
  TargetLineCalc_20ms/11(LCKLineC0) -> Bus Creator1/5
  Signal Copy15/1 -> Terminator33/1  "LSM_RFM_LineR1_C3"
  TargetLineCalc_20ms/18(HWARange) -> Bus Creator2/6
  TargetLineCalc_20ms/9(LCKLineC2) -> Bus Creator1/3
  Bus Selector3/5 -> TargetLineCalc_20ms/23(pathPredC0)  "<dC0V>"
  Bus Selector6/6 -> Signal Copy12/1  "<dDisStart>"
  TargetLineCalc_20ms/3(TJALineC2) -> Bus Creator/3
  Bus Selector4/1 -> TargetLineCalc_20ms/15(ACCMode)  "<ACC_ModeDisp>"
  Bus Selector5/6 -> Signal Copy5/1  "<dDisStart>"
  Bus Selector6/7 -> Signal Copy13/1  "<dDisFront>"
  Selector7/1 -> TargetLineCalc_20ms/12(EQ4_LRE_ELEM1)
  Bus Selector5/7 -> Signal Copy6/1  "<dDisFront>"
  TargetLineCalc_20ms/6(TJARange) -> Bus Creator/6
  RFM_LINE_L2/1 -> TargetLineCalc_20ms/38(RFM_LINE_L2)
  [LSM_LCK] -> LSM_Signal/2(In2)  "LSM_LCK"
  Constant1/1 -> Terminator2/1  "LSM_SubModel_Number"
  TargetLineCalc_20ms/40(MrcStopLane) -> Bus Creator2/28
  [LSM_UpdateCnt] -> LSM_Signal/5(In5)  "LSM_UpdateCnt"
  Signal Copy19/1 -> Terminator30/1  "LSM_RFM_LineR1_C0"
  TargetLineCalc_20ms/62(ESSRiRange) -> Bus Creator3/18
  TargetLineCalc_20ms/29(HWARiLineC0) -> Bus Creator2/17
  vxvRefMs/1 -> TargetLineCalc_20ms/1(vRef)
  RFM_LINE_L3/1 -> Terminator21/1
  Bus Selector7/5 -> Signal Copy15/1  "<dC3V>"
  TargetLineCalc_20ms/7(LCKLineValid) -> Bus Creator1/1
  TargetLineCalc_20ms/51(ESSLeLineValid) -> Bus Creator3/7
  TargetLineCalc_20ms/39(MRiLane) -> Bus Creator2/27
  EQ4_LRE/1 -> Bus Selector2/1
  RFM_LEFT_LANE/1 -> Terminator15/1
  TargetLineCalc_20ms/53(ESSLeLineC2) -> Bus Creator3/9
  TargetLineCalc_20ms/20(HWALeLineC3) -> Bus Creator2/8
  Bus Selector5/3 -> Signal Copy2/1  "<dC1V>"
  RFM_LINE_L1_1/1 -> TargetLineCalc_20ms/36(RFM_LINE_L1)
  RFM_UpdateCnt/1 -> TargetLineCalc_20ms/24(pathPredCnt)
  Bus Creator3/1 -> LSM_ESS/1, [LSM_ESS]
  TargetLineCalc_20ms/48(ESSLineC1) -> Bus Creator3/4
  RFM_ROAD/1 -> TargetLineCalc_20ms/27(RFM_ROAD)
  TargetLineCalc_20ms/64(PilotTurnSwSts) -> LSM_PilotTurnSwSts/1
  TargetLineCalc_20ms/4(TJALineC1) -> Bus Creator/4
  RFM_REC_LANES/1 -> TargetLineCalc_20ms/35(RFM_REC_LANES)
  Signal Copy2/1 -> Terminator6/1  "LSM_RFM_LineCenter_C1"
  TargetLineCalc_20ms/1(TJALineValid) -> Bus Creator/1
  Bus Selector5/1 -> Signal Copy/1  "<bIsLineExist>"
  Bus Selector6/2 -> Signal Copy8/1  "<dC0V>"
  PLAN_ALC_Decision/1 -> TargetLineCalc_20ms/25(PLAN_ALC_Decision)
  Bus Selector6/1 -> Signal Copy7/1  "<bIsLineExist>"
  TargetLineCalc_20ms/67(TJALineSource) -> LSM_TJALineSource/1
  TargetLineCalc_20ms/57(ESSRiLineValid) -> Bus Creator3/13
  TargetLineCalc_20ms/33(dyDiff) -> Bus Creator2/21
  TargetLineCalc_20ms/16(HWALineC1) -> Bus Creator2/4
  EQ4_LA/1 -> Bus Selector1/1
  TargetLineCalc_20ms/5(TJALineC0) -> Bus Creator/5
  TargetLineCalc_20ms/44(RiLineLcAvailable) -> Bus Creator2/32
  TargetLineCalc_20ms/41(HWALeLineVirtual) -> Bus Creator2/29
  TargetLineCalc_20ms/38(RightLaneChange) -> Bus Creator2/26
  Bus Creator1/1 -> LSM_LCK/1, [LSM_LCK]
  Signal Copy13/1 -> Terminator22/1  "LSM_RFM_LineL1_Front"
  TargetLineCalc_20ms/23(HWALeLineC0) -> Bus Creator2/11
  Bus Selector6/5 -> Signal Copy11/1  "<dC3V>"
  TargetLineCalc_20ms/56(ESSLeRange) -> Bus Creator3/12
  TOS_P0_TARGET_LINE/1 -> TargetLineCalc_20ms/14(P0TargetLine)
  Bus Selector4/2 -> TargetLineCalc_20ms/16(HWASts)  "<HWASts>"
  Selector/1 -> TargetLineCalc_20ms/3(EQ4_LA_ELEM_0)
  Ground/1 -> LSM_PilotNohExitDist/1
  Signal Copy14/1 -> Terminator32/1  "LSM_RFM_LineR1_C2"
  Bus Selector2/2 -> TargetLineCalc_20ms/13(LRE_HDR)  "<EQ4_LRE_HDR>"
  TargetLineCalc_20ms/8(LCKLineC3) -> Bus Creator1/2
  Bus Creator2/1 -> LSM_HWA/1, [LSM_HWA]
  RFM_LINE_R2/1 -> TargetLineCalc_20ms/39(RFM_LINE_R2)
  TargetLineCalc_20ms/59(ESSRiLineC2) -> Bus Creator3/15
  TargetLineCalc_20ms/22(HWALeLineC1) -> Bus Creator2/10
  [LSM_TJA_ICA] -> LSM_Signal/1(In1)  "LSM_TJA_ICA"
  TargetLineCalc_20ms/26(HWARiLineC3) -> Bus Creator2/14
  Signal Copy17/1 -> Terminator29/1  "LSM_RFM_LineR1_Front"
  TargetLineCalc_20ms/32(DoubleLineLost_b) -> Bus Creator2/20
  TargetLineCalc_20ms/14(HWALineC3) -> Bus Creator2/2
  RFM_LINE_EXIT_CL/1 -> TargetLineCalc_20ms/32(RFM_LINE_EXIT_CL)
  TargetLineCalc_20ms/45(ESSLineValid) -> Bus Creator3/1

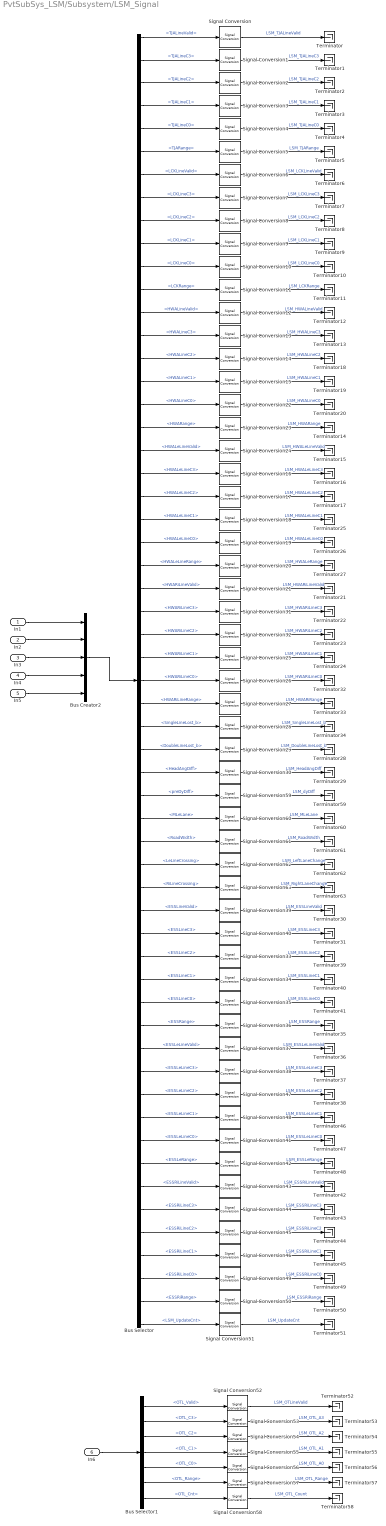
== system PvtSubSys_LSM/Subsystem/LSM_Signal ==
  In1 : Inport
  In2 : Inport  Port=2
  In3 : Inport  Port=3
  In4 : Inport  Port=4
  In5 : Inport  Port=5
  In6 : Inport  Port=6
  Bus Creator2 : BusCreator  Inputs=5
  Bus Selector : BusSelector  OutputSignals=LSM_TJA_ICA.TJALineValid,LSM_TJA_ICA.TJALineC3,LSM_TJA_ICA.TJALineC2,LSM_TJA_ICA.TJALineC1,LSM_TJA_ICA.TJALineC0,LSM_TJA_ICA.TJARange,LSM_LCK.LCKLineValid,LSM_LCK.LCKLineC3,LSM_LCK.LCKLineC2,LSM_LCK.LCKLineC1,LSM_LCK.LCKLineC0,LSM_LCK.LCKRange,LSM_HWA.HWALineValid,LSM_HWA.HWALineC3,LSM_HWA.HWALineC2,LSM_HWA.HWALineC1,LSM_HWA.HWALineC0,LSM_HWA.HWARange,LSM_HWA.HWALeLineValid,LSM_HWA.HWALeLineC3,LSM_HWA.HWALeLineC2,LSM_HWA.HWALeLineC1,LSM_HWA.HWALeLineC0,LSM_HWA.HWALeLineRange,LSM_HWA.HWARiLineValid,LSM_HWA.HWARiLineC3,LSM_HWA.HWARiLineC2,LSM_HWA.HWARiLineC1,LSM_HWA.HWARiLineC0,LSM_HWA.HWARiLineRange,LSM_HWA.SingleLineLost_b,LSM_HWA.DoubleLineLost_b,LSM_HWA.HeadAngDiff,LSM_HWA.preDyDiff,LSM_HWA.MLeLane,LSM_HWA.RoadWidth,LSM_HWA.LeLineCrossing,LSM_HWA.RiLineCrossing,LSM_ESS.ESSLineValid,LSM_ESS.ESSLineC3,LSM_ESS.ESSLineC2,LSM_ESS.ESSLineC1,LSM_ESS.ESSLineC0,LSM_ESS.ESSRange,LSM_ESS.ESSLeLineValid,LSM_ESS.ESSLeLineC3,LSM_ESS.ESSLeLineC2,LSM_ESS.ESSLeLineC1,LSM_ESS.ESSLeLineC0,LSM_ESS.ESSLeRange,LSM_ESS.ESSRiLineValid,LSM_ESS.ESSRiLineC3,LSM_ESS.ESSRiLineC2,LSM_ESS.ESSRiLineC1,LSM_ESS.ESSRiLineC0,LSM_ESS.ESSRiRange,LSM_UpdateCnt
  Bus Selector1 : BusSelector  OutputSignals=OTL_Valid,OTL_C3,OTL_C2,OTL_C1,OTL_C0,OTL_Range,OTL_Cnt
  Signal Conversion{,1..63} (64 alike) : SignalConversion  OverrideOpt=off
  Terminator{,1..63} (64 alike) : Terminator
  wires:
  In2/1 -> Bus Creator2/2
  Bus Creator2/1 -> Bus Selector/1
  In1/1 -> Bus Creator2/1
  Bus Selector/1 -> Signal Conversion/1  "<TJALineValid>"
  Signal Conversion/1 -> Terminator/1  "LSM_TJALineValid"
  In3/1 -> Bus Creator2/3
  In4/1 -> Bus Creator2/4
  In5/1 -> Bus Creator2/5
  Signal Conversion1/1 -> Terminator1/1  "LSM_TJALineC3"
  Bus Selector/2 -> Signal Conversion1/1  "<TJALineC3>"
  Bus Selector/3 -> Signal Conversion2/1  "<TJALineC2>"
  Signal Conversion2/1 -> Terminator2/1  "LSM_TJALineC2"
  Bus Selector/4 -> Signal Conversion3/1  "<TJALineC1>"
  Signal Conversion3/1 -> Terminator3/1  "LSM_TJALineC1"
  Bus Selector/5 -> Signal Conversion4/1  "<TJALineC0>"
  Bus Selector/6 -> Signal Conversion5/1  "<TJARange>"
  Bus Selector/7 -> Signal Conversion6/1  "<LCKLineValid>"
  Signal Conversion4/1 -> Terminator4/1  "LSM_TJALineC0"
  Signal Conversion5/1 -> Terminator5/1  "LSM_TJARange"
  Signal Conversion6/1 -> Terminator6/1  "LSM_LCKLineValid"
  Bus Selector/8 -> Signal Conversion7/1  "<LCKLineC3>"
  Bus Selector/9 -> Signal Conversion8/1  "<LCKLineC2>"
  Bus Selector/10 -> Signal Conversion9/1  "<LCKLineC1>"
  Bus Selector/11 -> Signal Conversion10/1  "<LCKLineC0>"
  Bus Selector/12 -> Signal Conversion11/1  "<LCKRange>"
  Bus Selector/13 -> Signal Conversion12/1  "<HWALineValid>"
  Bus Selector/14 -> Signal Conversion13/1  "<HWALineC3>"
  Bus Selector/15 -> Signal Conversion14/1  "<HWALineC2>"
  Bus Selector/16 -> Signal Conversion15/1  "<HWALineC1>"
  Bus Selector/17 -> Signal Conversion22/1  "<HWALineC0>"
  Bus Selector/18 -> Signal Conversion23/1  "<HWARange>"
  Bus Selector/19 -> Signal Conversion24/1  "<HWALeLineValid>"
  Bus Selector/20 -> Signal Conversion16/1  "<HWALeLineC3>"
  Bus Selector/21 -> Signal Conversion17/1  "<HWALeLineC2>"
  Bus Selector/22 -> Signal Conversion18/1  "<HWALeLineC1>"
  Bus Selector/23 -> Signal Conversion19/1  "<HWALeLineC0>"
  Bus Selector/24 -> Signal Conversion20/1  "<HWALeLineRange>"
  Bus Selector/25 -> Signal Conversion21/1  "<HWARiLineValid>"
  Bus Selector/26 -> Signal Conversion31/1  "<HWARiLineC3>"
  Bus Selector/27 -> Signal Conversion32/1  "<HWARiLineC2>"
  Bus Selector/28 -> Signal Conversion25/1  "<HWARiLineC1>"
  Bus Selector/29 -> Signal Conversion26/1  "<HWARiLineC0>"
  Bus Selector/30 -> Signal Conversion27/1  "<HWARiLineRange>"
  Bus Selector/31 -> Signal Conversion28/1  "<SingleLineLost_b>"
  Bus Selector/32 -> Signal Conversion29/1  "<DoubleLineLost_b>"
  Bus Selector/33 -> Signal Conversion30/1  "<HeadAngDiff>"
  Bus Selector/39 -> Signal Conversion39/1  "<ESSLineValid>"
  Bus Selector/40 -> Signal Conversion40/1  "<ESSLineC3>"
  Bus Selector/41 -> Signal Conversion33/1  "<ESSLineC2>"
  Bus Selector/42 -> Signal Conversion34/1  "<ESSLineC1>"
  Bus Selector/43 -> Signal Conversion35/1  "<ESSLineC0>"
  Bus Selector/44 -> Signal Conversion36/1  "<ESSRange>"
  Bus Selector/45 -> Signal Conversion37/1  "<ESSLeLineValid>"
  Bus Selector/46 -> Signal Conversion38/1  "<ESSLeLineC3>"
  Bus Selector/47 -> Signal Conversion47/1  "<ESSLeLineC2>"
  Bus Selector/48 -> Signal Conversion48/1  "<ESSLeLineC1>"
  Bus Selector/49 -> Signal Conversion41/1  "<ESSLeLineC0>"
  Bus Selector/50 -> Signal Conversion42/1  "<ESSLeRange>"
  Bus Selector/51 -> Signal Conversion43/1  "<ESSRiLineValid>"
  Bus Selector/52 -> Signal Conversion44/1  "<ESSRiLineC3>"
  Bus Selector/53 -> Signal Conversion45/1  "<ESSRiLineC2>"
  Bus Selector/54 -> Signal Conversion46/1  "<ESSRiLineC1>"
  Bus Selector/55 -> Signal Conversion49/1  "<ESSRiLineC0>"
  Bus Selector/56 -> Signal Conversion50/1  "<ESSRiRange>"
  Bus Selector/57 -> Signal Conversion51/1  "<LSM_UpdateCnt>"
  Signal Conversion7/1 -> Terminator7/1  "LSM_LCKLineC3"
  Signal Conversion8/1 -> Terminator8/1  "LSM_LCKLineC2"
  Signal Conversion9/1 -> Terminator9/1  "LSM_LCKLineC1"
  Signal Conversion10/1 -> Terminator10/1  "LSM_LCKLineC0"
  Signal Conversion11/1 -> Terminator11/1  "LSM_LCKRange"
  Signal Conversion12/1 -> Terminator12/1  "LSM_HWALineValid"
  Signal Conversion13/1 -> Terminator13/1  "LSM_HWALineC3"
  Signal Conversion14/1 -> Terminator18/1  "LSM_HWALineC2"
  Signal Conversion15/1 -> Terminator19/1  "LSM_HWALineC1"
  Signal Conversion22/1 -> Terminator20/1  "LSM_HWALineC0"
  Signal Conversion23/1 -> Terminator14/1  "LSM_HWARange"
  Signal Conversion24/1 -> Terminator15/1  "LSM_HWALeLineValid"
  Signal Conversion16/1 -> Terminator16/1  "LSM_HWALeLineC3"
  Signal Conversion17/1 -> Terminator17/1  "LSM_HWALeLineC2"
  Signal Conversion18/1 -> Terminator25/1  "LSM_HWALeLineC1"
  Signal Conversion19/1 -> Terminator26/1  "LSM_HWALeLineC0"
  Signal Conversion20/1 -> Terminator27/1  "LSM_HWALeRange"
  Signal Conversion21/1 -> Terminator21/1  "LSM_HWARiLineValid"
  Signal Conversion31/1 -> Terminator22/1  "LSM_HWARiLineC3"
  Signal Conversion32/1 -> Terminator23/1  "LSM_HWARiLineC2"
  Signal Conversion25/1 -> Terminator24/1  "LSM_HWARiLineC1"
  Signal Conversion26/1 -> Terminator32/1  "LSM_HWARiLineC0"
  Signal Conversion27/1 -> Terminator33/1  "LSM_HWARiRange"
  Signal Conversion28/1 -> Terminator34/1  "LSM_SingleLineLost_b"
  Signal Conversion29/1 -> Terminator28/1  "LSM_DoubleLineLost_b"
  Signal Conversion30/1 -> Terminator29/1  "LSM_HeadAngDiff"
  Signal Conversion39/1 -> Terminator30/1  "LSM_ESSLineValid"
  Signal Conversion40/1 -> Terminator31/1  "LSM_ESSLineC3"
  Signal Conversion33/1 -> Terminator39/1  "LSM_ESSLineC2"
  Signal Conversion34/1 -> Terminator40/1  "LSM_ESSLineC1"
  Signal Conversion35/1 -> Terminator41/1  "LSM_ESSLineC0"
  Signal Conversion36/1 -> Terminator35/1  "LSM_ESSRange"
  Signal Conversion37/1 -> Terminator36/1  "LSM_ESSLeLineValid"
  Signal Conversion38/1 -> Terminator37/1  "LSM_ESSLeLineC3"
  Signal Conversion47/1 -> Terminator38/1  "LSM_ESSLeLineC2"
  Signal Conversion48/1 -> Terminator46/1  "LSM_ESSLeLineC1"
  Signal Conversion41/1 -> Terminator47/1  "LSM_ESSLeLineC0"
  Signal Conversion42/1 -> Terminator48/1  "LSM_ESSLeRange"
  Signal Conversion43/1 -> Terminator42/1  "LSM_ESSRiLineValid"
  Signal Conversion44/1 -> Terminator43/1  "LSM_ESSRiLineC3"
  Signal Conversion45/1 -> Terminator44/1  "LSM_ESSRiLineC2"
  Signal Conversion46/1 -> Terminator45/1  "LSM_ESSRiLineC1"
  Signal Conversion49/1 -> Terminator49/1  "LSM_ESSRiLineC0"
  Signal Conversion50/1 -> Terminator50/1  "LSM_ESSRiRange"
  Signal Conversion51/1 -> Terminator51/1  "LSM_UpdateCnt"
  Signal Conversion57/1 -> Terminator57/1  "LSM_OTL_Range"
  Signal Conversion56/1 -> Terminator56/1  "LSM_OTL_A0"
  Bus Selector1/5 -> Signal Conversion56/1  "<OTL_C0>"
  Signal Conversion58/1 -> Terminator58/1  "LSM_OTL_Count"
  Signal Conversion55/1 -> Terminator55/1  "LSM_OTL_A1"
  Bus Selector1/4 -> Signal Conversion55/1  "<OTL_C1>"
  Bus Selector1/2 -> Signal Conversion53/1  "<OTL_C3>"
  Signal Conversion54/1 -> Terminator54/1  "LSM_OTL_A2"
  Bus Selector1/7 -> Signal Conversion58/1  "<OTL_Cnt>"
  Bus Selector1/6 -> Signal Conversion57/1  "<OTL_Range>"
  In6/1 -> Bus Selector1/1
  Signal Conversion53/1 -> Terminator53/1  "LSM_OTL_A3"
  Signal Conversion52/1 -> Terminator52/1  "LSM_OTLineValid"
  Bus Selector1/3 -> Signal Conversion54/1  "<OTL_C2>"
  Bus Selector1/1 -> Signal Conversion52/1  "<OTL_Valid>"
  Bus Selector/34 -> Signal Conversion59/1  "<preDyDiff>"
  Bus Selector/35 -> Signal Conversion60/1  "<MLeLane>"
  Bus Selector/36 -> Signal Conversion61/1  "<RoadWidth>"
  Signal Conversion61/1 -> Terminator61/1  "LSM_RoadWidth"
  Signal Conversion60/1 -> Terminator60/1  "LSM_MLeLane"
  Signal Conversion59/1 -> Terminator59/1  "LSM_dyDiff"
  Bus Selector/37 -> Signal Conversion62/1  "<LeLineCrossing>"
  Bus Selector/38 -> Signal Conversion63/1  "<RiLineCrossing>"
  Signal Conversion62/1 -> Terminator62/1  "LSM_LeftLaneChange"
  Signal Conversion63/1 -> Terminator63/1  "LSM_RightLaneChange"
